simulink model "UDPM_in"  (R2018b)
settings: Solver=FixedStepDiscrete  StartTime=0.0  StopTime=inf  FixedStep=0.001  RelTol=1e-3
undefined symbols (not defined in the file): f, selecting_parameters
libraries: etargetslib x1, instrumentlib x1
settings Model: Creator=Daniele Nava  LastModifiedBy=Daniele Nava

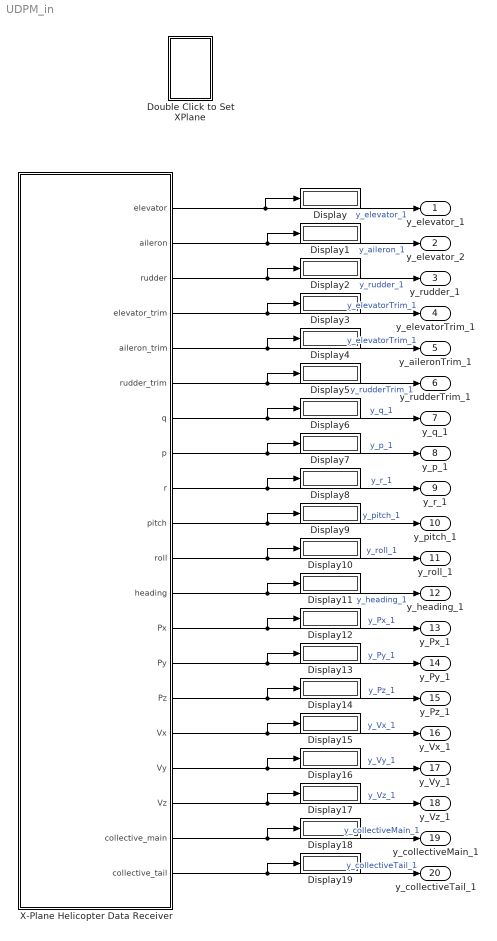
== system UDPM_in ==
  Display{,1..19} (20 alike) : Display
  Double Click to Set XPlane : Subsystem  LoadFcn=selecting_parameters()
      settings: OpenFcn=selecting_parameters()
  X-Plane Helicopter Data Receiver : Subsystem  AncestorBlock=X_Plane_Communication_Library/Helicopter/X-Plane Helicopter Data Receiver  mask{ip_adress='127.0.0.1', port_number=49004}
      mask prompts: ip_adress "Local IP Adress (default: '127.0.0.1')"; port_number "Input Port Number (default: '49004')"
      mask help: This block is configured to receive data to an helicopter aircraft on X-Plane Flight Simulator.
      mask Help: Contact adrianobittar@gmail.com
  y_elevator_1 : Outport
  y_elevator_2 : Outport  Port=2
  y_rudder_1 : Outport  Port=3
  y_elevatorTrim_1 : Outport  Port=4
  y_aileronTrim_1 : Outport  Port=5
  y_rudderTrim_1 : Outport  Port=6
  y_q_1 : Outport  Port=7
  y_p_1 : Outport  Port=8
  y_r_1 : Outport  Port=9
  y_pitch_1 : Outport  Port=10
  y_roll_1 : Outport  Port=11
  y_heading_1 : Outport  Port=12
  y_Px_1 : Outport  Port=13
  y_Py_1 : Outport  Port=14
  y_Pz_1 : Outport  Port=15
  y_Vx_1 : Outport  Port=16
  y_Vy_1 : Outport  Port=17
  y_Vz_1 : Outport  Port=18
  y_collectiveMain_1 : Outport  Port=19
  y_collectiveTail_1 : Outport  Port=20
  wires:
  X-Plane Helicopter Data Receiver/1("elevator ") -> y_elevator_1/1, Display/1  "y_elevator_1"
  X-Plane Helicopter Data Receiver/2(aileron) -> y_elevator_2/1, Display1/1  "y_aileron_1"
  X-Plane Helicopter Data Receiver/3(rudder) -> y_rudder_1/1, Display2/1  "y_rudder_1"
  X-Plane Helicopter Data Receiver/4(elevator_trim) -> y_elevatorTrim_1/1, Display3/1  "y_elevatorTrim_1"
  X-Plane Helicopter Data Receiver/5(aileron_trim) -> y_aileronTrim_1/1, Display4/1  "y_elevatorTrim_1"
  X-Plane Helicopter Data Receiver/8(p) -> y_p_1/1, Display7/1  "y_p_1"
  X-Plane Helicopter Data Receiver/7(q) -> y_q_1/1, Display6/1  "y_q_1"
  X-Plane Helicopter Data Receiver/6(rudder_trim) -> y_rudderTrim_1/1, Display5/1  "y_rudderTrim_1"
  X-Plane Helicopter Data Receiver/15(Pz) -> y_Pz_1/1, Display14/1  "y_Pz_1"
  X-Plane Helicopter Data Receiver/14(Py) -> y_Py_1/1, Display13/1  "y_Py_1"
  X-Plane Helicopter Data Receiver/13(Px) -> y_Px_1/1, Display12/1  "y_Px_1"
  X-Plane Helicopter Data Receiver/9(r) -> y_r_1/1, Display8/1  "y_r_1"
  X-Plane Helicopter Data Receiver/12(heading) -> y_heading_1/1, Display11/1  "y_heading_1"
  X-Plane Helicopter Data Receiver/11(roll) -> y_roll_1/1, Display10/1  "y_roll_1"
  X-Plane Helicopter Data Receiver/16(Vx) -> y_Vx_1/1, Display15/1  "y_Vx_1"
  X-Plane Helicopter Data Receiver/10(pitch) -> y_pitch_1/1, Display9/1  "y_pitch_1"
  X-Plane Helicopter Data Receiver/18(Vz) -> y_Vz_1/1, Display17/1  "y_Vz_1"
  X-Plane Helicopter Data Receiver/19(collective_main) -> y_collectiveMain_1/1, Display18/1  "y_collectiveMain_1"
  X-Plane Helicopter Data Receiver/20(collective_tail) -> y_collectiveTail_1/1, Display19/1  "y_collectiveTail_1"
  X-Plane Helicopter Data Receiver/17(Vy) -> y_Vy_1/1, Display16/1  "y_Vy_1"

== system UDPM_in/Double Click to Set XPlane ==

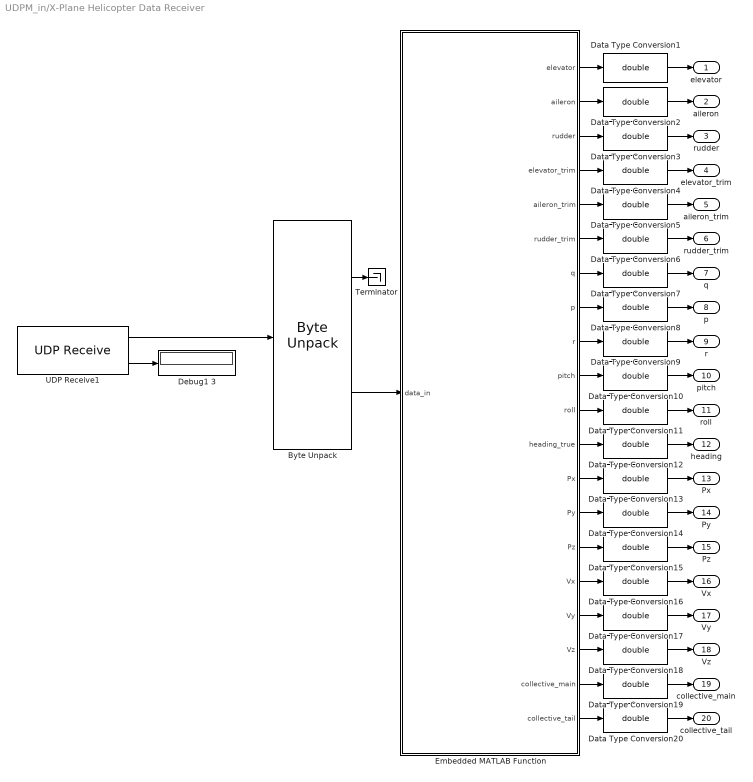
== system UDPM_in/X-Plane Helicopter Data Receiver ==
  Byte Unpack : etargetslib/Byte Unpack  dimensions={5,[9,6]}  datatypes={'uint8','single'}  byteAlign=1
  Data Type Conversion{1..20} (20 alike) : DataTypeConversion  OutDataTypeStr=double  SaturateOnIntegerOverflow=on
  Debug1 3 : Display
  Embedded MATLAB Function : MATLAB Function  TreatAsAtomicUnit=on
  Terminator : Terminator
  UDP Receive1 : instrumentlib/UDP Receive  Host=127.0.0.1  Port=50001  LocalPort=50001  EnablePortSharing=on  GetLatestData=off  DataSize=[1 1]  DataType=uint8  ASCIIFormatting=%f,  Terminator=LF  ByteOrder=BigEndian  EnableBlockingMode=off  Timeout=10  SampleTime=0.01  LocalAddress=127.0.0.1
      settings: SourceProductName=Instrument Control Toolbox
  "elevator " : Outport
  aileron : Outport  Port=2
  rudder : Outport  Port=3
  elevator_trim : Outport  Port=4
  aileron_trim : Outport  Port=5
  rudder_trim : Outport  Port=6
  q : Outport  Port=7
  p : Outport  Port=8
  r : Outport  Port=9
  pitch : Outport  Port=10
  roll : Outport  Port=11
  heading : Outport  Port=12
  Px : Outport  Port=13
  Py : Outport  Port=14
  Pz : Outport  Port=15
  Vx : Outport  Port=16
  Vy : Outport  Port=17
  Vz : Outport  Port=18
  collective_main : Outport  Port=19
  collective_tail : Outport  Port=20
  wires:
  Byte Unpack/2 -> Embedded MATLAB Function/1(data_in)
  Data Type Conversion20/1 -> collective_tail/1
  Data Type Conversion7/1 -> q/1
  Embedded MATLAB Function/9(r) -> Data Type Conversion9/1
  Embedded MATLAB Function/15(Pz) -> Data Type Conversion15/1
  Data Type Conversion3/1 -> rudder/1
  Embedded MATLAB Function/16(Vx) -> Data Type Conversion16/1
  Embedded MATLAB Function/2(aileron) -> Data Type Conversion2/1
  Embedded MATLAB Function/17(Vy) -> Data Type Conversion17/1
  Data Type Conversion14/1 -> Py/1
  Embedded MATLAB Function/4(elevator_trim) -> Data Type Conversion4/1
  Data Type Conversion17/1 -> Vy/1
  Embedded MATLAB Function/13(Px) -> Data Type Conversion13/1
  Embedded MATLAB Function/12(heading_true) -> Data Type Conversion12/1
  Data Type Conversion16/1 -> Vx/1
  Embedded MATLAB Function/20(collective_tail) -> Data Type Conversion20/1
  Embedded MATLAB Function/6(rudder_trim) -> Data Type Conversion6/1
  Embedded MATLAB Function/19(collective_main) -> Data Type Conversion19/1
  Embedded MATLAB Function/5(aileron_trim) -> Data Type Conversion5/1
  Embedded MATLAB Function/14(Py) -> Data Type Conversion14/1
  Data Type Conversion19/1 -> collective_main/1
  Data Type Conversion15/1 -> Pz/1
  Data Type Conversion5/1 -> aileron_trim/1
  Data Type Conversion18/1 -> Vz/1
  Embedded MATLAB Function/18(Vz) -> Data Type Conversion18/1
  Embedded MATLAB Function/7(q) -> Data Type Conversion7/1
  Data Type Conversion11/1 -> roll/1
  Data Type Conversion9/1 -> r/1
  Data Type Conversion6/1 -> rudder_trim/1
  Data Type Conversion2/1 -> aileron/1
  Embedded MATLAB Function/3(rudder) -> Data Type Conversion3/1
  Data Type Conversion10/1 -> pitch/1
  Embedded MATLAB Function/1(elevator) -> Data Type Conversion1/1
  Embedded MATLAB Function/11(roll) -> Data Type Conversion11/1
  Data Type Conversion12/1 -> heading/1
  Embedded MATLAB Function/8(p) -> Data Type Conversion8/1
  Data Type Conversion4/1 -> elevator_trim/1
  Byte Unpack/1 -> Terminator/1
  Data Type Conversion1/1 -> "elevator "/1
  Data Type Conversion13/1 -> Px/1
  Data Type Conversion8/1 -> p/1
  Embedded MATLAB Function/10(pitch) -> Data Type Conversion10/1
  UDP Receive1/2 -> Debug1 3/1
  UDP Receive1/1 -> Byte Unpack/1

== matlab function UDPM_in/X-Plane Helicopter Data Receiver/Embedded MATLAB Function ==
  data: data_in input; elevator output; aileron output; rudder output; elevator_trim output; aileron_trim output; rudder_trim output; q output; p output; r output; pitch output; roll output; heading_true output; Px output; Py output; Pz output; Vx output; Vy output; Vz output; collective_main output; collective_tail output
function [elevator, aileron, rudder, elevator_trim, aileron_trim, rudder_trim, q,p,r, pitch, roll, heading_true, Px, Py, Pz, Vx, Vy, Vz, collective_main, collective_tail]   = fcn(data_in)
% This block supports the Embedded MATLAB subset.
% See the help menu for details. 

elevator = data_in(2,1);
aileron = data_in(3,1);
rudder= data_in(4,1);


elevator_trim= data_in(2,2);
aileron_trim= data_in(3,2);
rudder_trim= data_in(4,2);

q= data_in(2,3);
p= data_in(3,3);
r= data_in(4,3);

pitch= data_in(2,4);
roll= data_in(3,4);
heading_true= data_in(4,4);

Px= data_in(2,5);
Py= data_in(3,5);
Pz= data_in(4,5);
Vx= data_in(5,5);
Vy= data_in(6,5);
Vz= data_in(7,5);

collective_main= data_in(2,6);
collective_tail= data_in(3,6);
